simulink model "Problem6_DirectForm_ReferenceModel"  (R2020b)
settings: Solver=VariableStepAuto  StartTime=0.0  StopTime=10.0  RelTol=1e-3
settings Model: Creator=vigne  LastModifiedBy=vigne
settings DataIOCC: SaveOutput=off  SaveTime=off

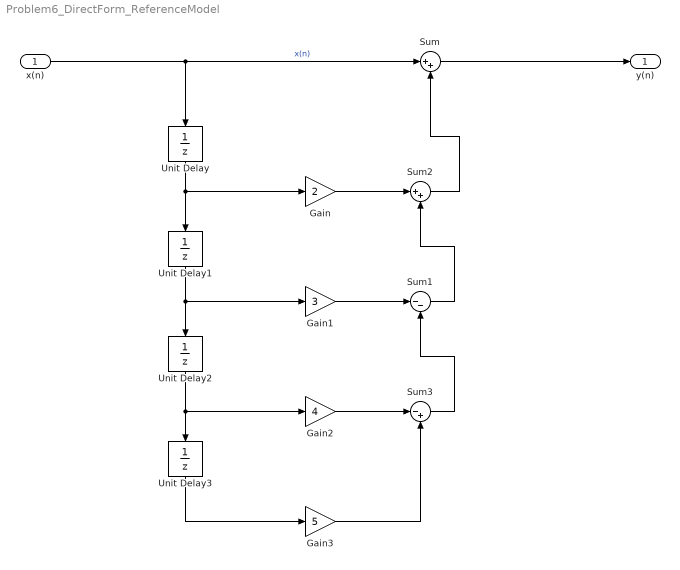
== system Problem6_DirectForm_ReferenceModel ==
  x(n) : Inport  OutDataTypeStr=double  PortDimensions=1  SampleTime=0
  Gain : Gain  Gain=2
  Gain1 : Gain  Gain=3
  Gain2 : Gain  Gain=4
  Gain3 : Gain  Gain=5
  Sum : Sum  Inputs=|++
  Sum1 : Sum  Inputs=|--
  Sum2 : Sum  Inputs=|++
  Sum3 : Sum  Inputs=|-+
  Unit Delay{,1..3} (4 alike) : UnitDelay  SampleTime=-1  HasFrameUpgradeWarning=on
  y(n) : Outport  OutDataTypeStr=double  PortDimensions=1  SampleTime=0
  wires:
  Sum2/1 -> Sum/2
  Sum1/1 -> Sum2/2
  x(n)/1 -> Unit Delay/1, Sum/1  "x(n)"
  Gain2/1 -> Sum3/1
  Unit Delay1/1 -> Unit Delay2/1, Gain1/1
  Unit Delay3/1 -> Gain3/1
  Unit Delay2/1 -> Unit Delay3/1, Gain2/1
  Gain1/1 -> Sum1/1
  Unit Delay/1 -> Gain/1, Unit Delay1/1
  Gain/1 -> Sum2/1
  Sum3/1 -> Sum1/2
  Gain3/1 -> Sum3/2
  Sum/1 -> y(n)/1
